simulink model "Hinf_Arduino"  (R2025b)
settings: Solver=FixedStepDiscrete  StartTime=0.0  StopTime=Inf  FixedStep=Ts_SMC_Arduino  RelTol=1e-3  EnableMultiTasking=on
InitFcn:
  | Ts_hinf = 0.01;
  | Ts_SMC_Arduino  = Ts_hinf;
  | Ts_MRAC_Arduino = Ts_hinf;
  | 
  | u0_eq = 35.1444323672;
  | 
  | control_enable_SMC = 1;
  | u_min_MRAC = 0;
  | u_max_MRAC = 100;
  | 
  | gyro_bias_dps_SMC = 0;
  | gyro_sign_SMC     = 1;
undefined symbols (not defined in the file or in its folder): dspblkCoreblockFVToolHelper, gcbh
libraries: arduinolib x2, arduinosensorlib x1
settings Model: ExtModeTrigDuration=2  Creator=juanm  LastModifiedBy=nicao
settings SolverCC: AutoInsertRateTranBlk=on
settings OptimizationCC: EnhancedBackFolding=on  PassReuseOutputArgsThreshold=0.0  MaxStackSize=64  OptimizeBlockOrder=speed  DifferentSizesBufferReuse=on  OptimizationCustomize=off
settings DebuggingCC: ParameterTunabilityLossMsg=error
settings HardwareCC: ProdBitPerInt=16.0  ProdBitPerPointer=16.0  ProdBitPerSizeT=16.0  ProdBitPerPtrDiffT=16.0  ProdLargestAtomicFloat=None  ProdWordSize=8.0  ProdHWDeviceType=Atmel->AVR  UseEmbeddedCoderFeatures=off  UseSimulinkCoderFeatures=off
settings SFSimCC: MATLABDynamicMemAlloc=off
settings RTWCC: SystemTargetFile=ert.tlc  HardwareBoard=Arduino Uno  TemplateMakefile=ert_default_tmf  Toolchain=Arduino AVR  BuildConfiguration=Faster Runs  Description=Embedded Coder
settings CodeAppCC: ForceParamTrailComments=on  OperatorAnnotations=on
settings ERTTargetCC: ExtModeTransport=3.0  ExtModeStaticAlloc=on  ExtModeAutomaticAllocSize=off  ExtModeStaticAllocSize=250.0  ExtModeMexFile=ext_xcp  ExtModeIntrfLevel=Level2 - Open  InlinedParameterPlacement=Hierarchical  ERTCustomFileBanners=off  SupportContinuousTime=on  SupportNonInlinedSFcns=on  RemoveResetFunc=off  SupportVariableSizeSignals=on  ModelStepFunctionPrototypeControlCompliant=off

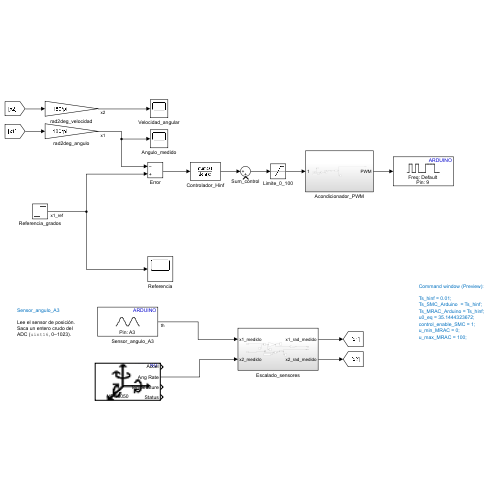
[thumbnail: Simulink's stored preview of the top-level diagram]
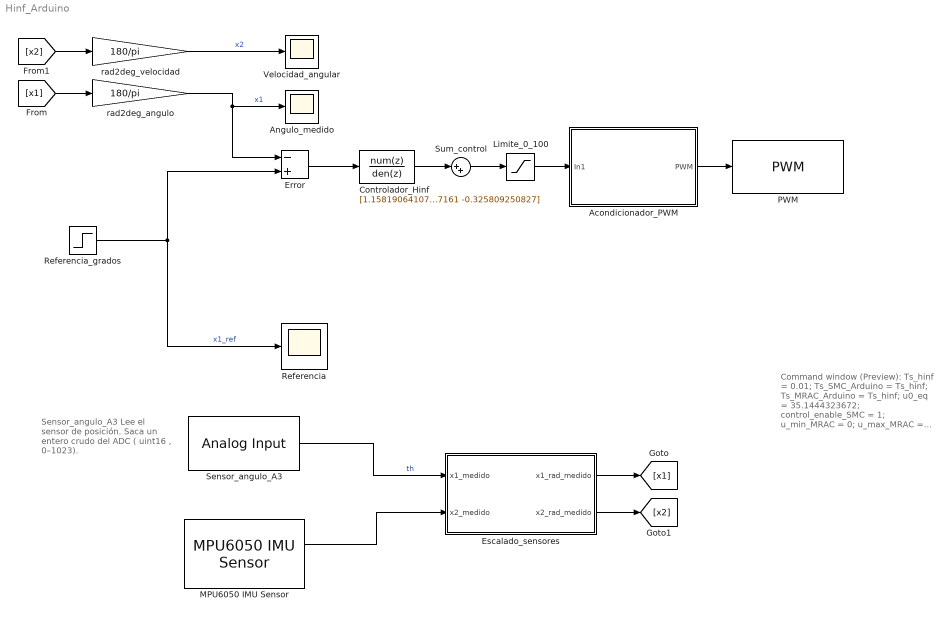
== system Hinf_Arduino ==
  note: Sensor_angulo_A3
      |
      | Lee el sensor de posición. Saca un entero crudo del ADC ( uint16 , 0–1023).
  note: Command window (Preview):
      |
      | Ts_hinf = 0.01;
      | Ts_SMC_Arduino = Ts_hinf;
      | Ts_MRAC_Arduino = Ts_hinf;
      | u0_eq = 35.1444323672;
      | control_enable_SMC = 1;
      | u_min_MRAC = 0;
      | u_max_MRAC = 100;
  "\tSensor_angulo_A3" : arduinolib/Analog Input  pinNumber=3  ReadResultsOnly=off  ConversionTriggerSource=Software  ExternalTriggerType=uint32( 0 )  OutputDataType=uint16  EnableConversionCompleteNotify=off  EnableOuputStatus=off  SampleTime=-1  blockPlatform=arduino
  Acondicionador_PWM : Subsystem
  Angulo_medido : Scope
  Controlador_Hinf : DiscreteTransferFcn  LoadFcn=dspblkCoreblockFVToolHelper(gcbh,'load');  Numerator=[1.15819064107 -0.463870070534 -1.80823927917 0.469530856268 0.655709423838]  Denominator=[1 -1.54880027756 0.124342533919 0.750269557161 -0.325809250827]
      settings: CopyFcn=dspblkCoreblockFVToolHelper(gcbh,'copy');  DeleteFcn=dspblkCoreblockFVToolHelper(gcbh,'close');  ModelCloseFcn=dspblkCoreblockFVToolHelper(gcbh,'close');  PreSaveFcn=dspblkCoreblockFVToolHelper(gcbh,'presave');  PostSaveFcn=dspblkCoreblockFVToolHelper(gcbh,'postsave');  CloseFcn=dspblkCoreblockFVToolHelper(gcbh,'close');
  Error : Sum  Inputs=-+
  Escalado_sensores : Subsystem
  Limite_0_100 : Saturate  UpperLimit=100  LowerLimit=0  ZeroCross=off
  MPU6050 IMU Sensor : arduinosensorlib/MPU6050 IMU Sensor  I2CModule=0  SlaveAddress=0x69  Accel=on  AngularRate=on  Temperature=on  Status=on  Timestamp=off  EulerAngles=off  Quat=off  AccelRange=2G  GyroRange=250 dps  DmpOdr=200 Hz  Dlpf=Accelerometer: 184Hz, Gyroscope: 188Hz  spf=1  SampleTime=-1  QueueSizeFactor=1
  PWM : arduinolib/PWM  pinNumber=9  frequencyType=Default  desiredFrequency=490.2  achievableFrequency=490.2
  Referencia : Scope
  Referencia_grados : Step  After=110  SampleTime=0
  Sum_control : Sum  Inputs=|++
  Velocidad_angular : Scope
  rad2deg_angulo : Gain  Gain=180/pi
  rad2deg_velocidad : Gain  Gain=180/pi
  wires:
  "\tSensor_angulo_A3"/1 -> Escalado_sensores/1(x1_medido)  "th"
  Referencia_grados/1 -> Error/2, Referencia/1  "x1_ref"
  Escalado_sensores/2(x2_rad_medido) -> [x2]
  Escalado_sensores/1(x1_rad_medido) -> [x1]
  [x1] -> rad2deg_angulo/1
  [x2] -> rad2deg_velocidad/1
  rad2deg_angulo/1 -> Error/1, Angulo_medido/1  "x1"
  rad2deg_velocidad/1 -> Velocidad_angular/1  "x2"
  Error/1 -> Controlador_Hinf/1
  Sum_control/1 -> Limite_0_100/1
  Limite_0_100/1 -> Acondicionador_PWM/1(In1)
  Acondicionador_PWM/1(PWM) -> PWM/1
  Controlador_Hinf/1 -> Sum_control/1
  MPU6050 IMU Sensor/2 -> Escalado_sensores/2(x2_medido)

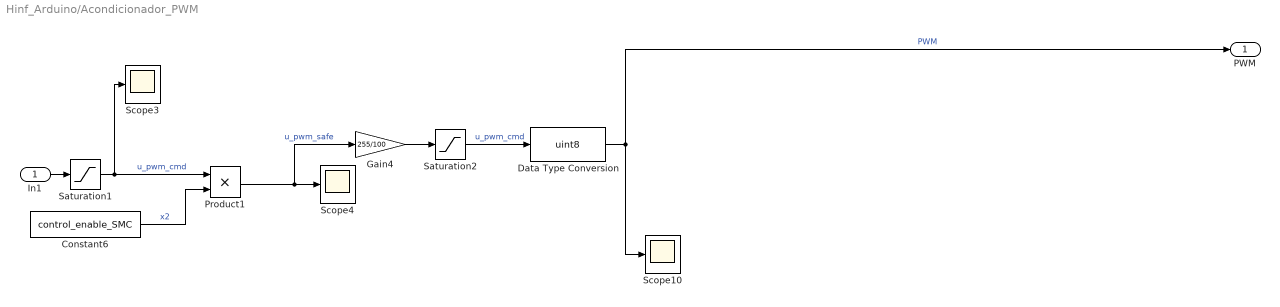
== system Hinf_Arduino/Acondicionador_PWM ==
  In1 : Inport
  Constant6 : Constant  Value=control_enable_SMC  VectorParams1D=off
  Data Type Conversion : DataTypeConversion  OutDataTypeStr=uint8  SaturateOnIntegerOverflow=off  RndMeth=Floor
  Gain4 : Gain  Gain=255/100
  Product1 : Product
  Saturation1 : Saturate  UpperLimit=u_max_MRAC  LowerLimit=u_min_MRAC
  Saturation2 : Saturate  UpperLimit=255  LowerLimit=0
  Scope10 : Scope
  Scope3 : Scope
  Scope4 : Scope
  PWM : Outport
  wires:
  Gain4/1 -> Saturation2/1
  Saturation1/1 -> Scope3/1, Product1/1  "u_pwm_cmd"
  Constant6/1 -> Product1/2  "x2"
  In1/1 -> Saturation1/1
  Saturation2/1 -> Data Type Conversion/1  "u_pwm_cmd"
  Product1/1 -> Gain4/1, Scope4/1  "u_pwm_safe"
  Data Type Conversion/1 -> PWM/1, Scope10/1  "PWM"

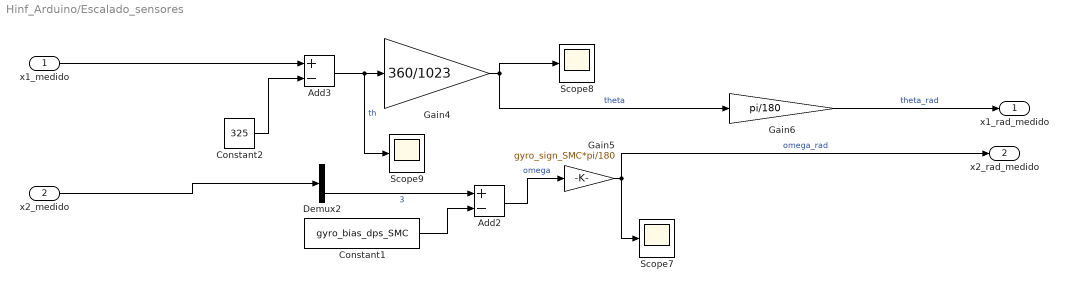
== system Hinf_Arduino/Escalado_sensores ==
  x1_medido : Inport
  x2_medido : Inport  Port=2
  Add2 : Sum  Inputs=+-
  Add3 : Sum  Inputs=+-
  Constant1 : Constant  Value=gyro_bias_dps_SMC
  Constant2 : Constant  Value=325
  Demux2 : Demux  Outputs=3
  Gain4 : Gain  Gain=360/1023
  Gain5 : Gain  Gain=gyro_sign_SMC*pi/180
  Gain6 : Gain  Gain=pi/180
  Scope7 : Scope
  Scope8 : Scope
  Scope9 : Scope
  x1_rad_medido : Outport
  x2_rad_medido : Outport  Port=2
  wires:
  Add3/1 -> Scope9/1, Gain4/1  "th"
  Gain6/1 -> x1_rad_medido/1  "theta_rad"
  Gain4/1 -> Gain6/1, Scope8/1  "theta"
  Demux2/3 -> Add2/1  "3"
  x1_medido/1 -> Add3/1
  Gain5/1 -> x2_rad_medido/1, Scope7/1  "omega_rad"
  Constant1/1 -> Add2/2
  x2_medido/1 -> Demux2/1
  Add2/1 -> Gain5/1  "omega"
  Constant2/1 -> Add3/2
